simulink model "TPS_failure_system2020"  (R2020a)
settings: Solver=VariableStepAuto  StartTime=0.0  StopTime=10.0  RelTol=1e-3
undefined symbols (not defined in the file or in its folder): APP_modes
libraries: simulink x5
settings Model: Creator=Administrator  LastModifiedBy=Administrator

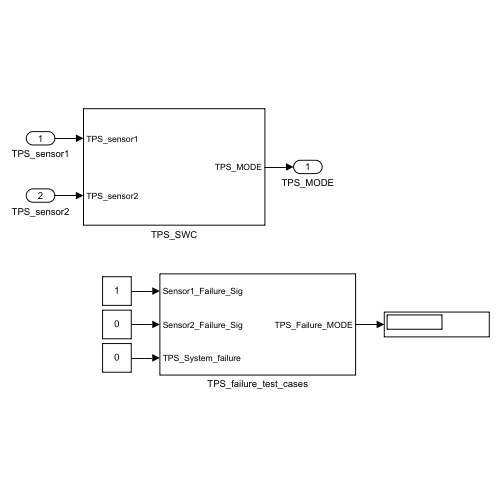
[thumbnail: Simulink's stored preview of the top-level diagram]
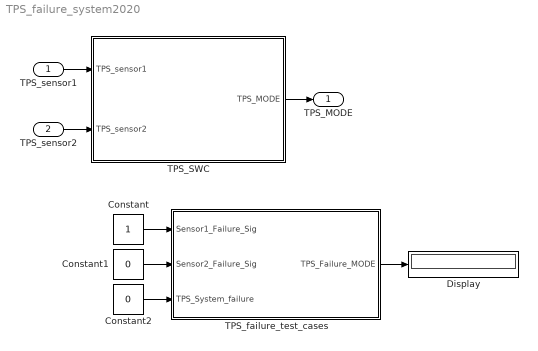
== system TPS_failure_system2020 ==
  TPS_sensor1 : Inport  OutDataTypeStr=single
  TPS_sensor2 : Inport  Port=2  OutDataTypeStr=single
  Constant : Constant  OutDataTypeStr=boolean
  Constant1 : Constant  Value=0  OutDataTypeStr=boolean
  Constant2 : Constant  Value=0  OutDataTypeStr=boolean
  Display : Display
  TPS_SWC : Subsystem
  TPS_failure_test_cases : Subsystem
  TPS_MODE : Outport
  wires:
  TPS_failure_test_cases/1(TPS_Failure_MODE) -> Display/1
  Constant/1 -> TPS_failure_test_cases/1(Sensor1_Failure_Sig)
  Constant1/1 -> TPS_failure_test_cases/2(Sensor2_Failure_Sig)
  Constant2/1 -> TPS_failure_test_cases/3(TPS_System_failure)
  TPS_SWC/1(TPS_MODE) -> TPS_MODE/1
  TPS_sensor1/1 -> TPS_SWC/1(TPS_sensor1)
  TPS_sensor2/1 -> TPS_SWC/2(TPS_sensor2)

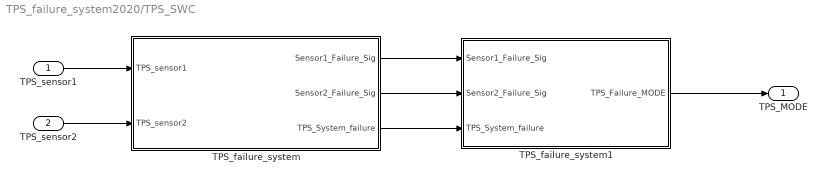
== system TPS_failure_system2020/TPS_SWC ==
  TPS_sensor1 : Inport  OutDataTypeStr=single
  TPS_sensor2 : Inport  Port=2  OutDataTypeStr=single
  TPS_failure_system : Subsystem
  TPS_failure_system1 : Subsystem
  TPS_MODE : Outport
  wires:
  TPS_failure_system/1(Sensor1_Failure_Sig) -> TPS_failure_system1/1(Sensor1_Failure_Sig)
  TPS_failure_system1/1(TPS_Failure_MODE) -> TPS_MODE/1
  TPS_sensor1/1 -> TPS_failure_system/1(TPS_sensor1)
  TPS_sensor2/1 -> TPS_failure_system/2(TPS_sensor2)
  TPS_failure_system/2(Sensor2_Failure_Sig) -> TPS_failure_system1/2(Sensor2_Failure_Sig)
  TPS_failure_system/3(TPS_System_failure) -> TPS_failure_system1/3(TPS_System_failure)

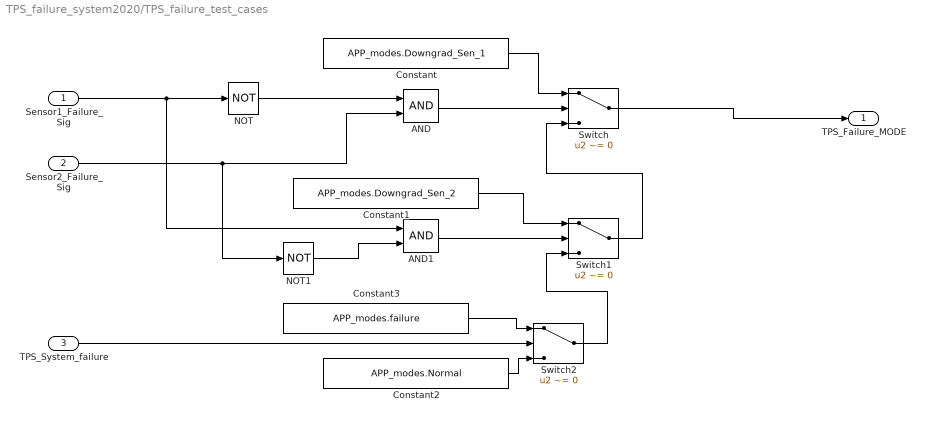
== system TPS_failure_system2020/TPS_failure_test_cases ==
  Sensor1_Failure_Sig : Inport  OutDataTypeStr=boolean
  Sensor2_Failure_Sig : Inport  Port=2  OutDataTypeStr=boolean
  TPS_System_failure : Inport  Port=3  OutDataTypeStr=boolean
  AND : Logic  AllPortsSameDT=off  OutDataTypeStr=boolean
  AND1 : Logic  AllPortsSameDT=off  OutDataTypeStr=boolean
  Constant : Constant  Value=APP_modes.Downgrad_Sen_1
  Constant1 : Constant  Value=APP_modes.Downgrad_Sen_2
  Constant2 : Constant  Value=APP_modes.Normal
  Constant3 : Constant  Value=APP_modes.failure
  NOT : Logic  Operator=NOT  IconShape=distinctive  AllPortsSameDT=off  OutDataTypeStr=boolean
  NOT1 : Logic  Operator=NOT  IconShape=distinctive  AllPortsSameDT=off  OutDataTypeStr=boolean
  Switch : Switch  Criteria=u2 ~= 0
  Switch1 : Switch  Criteria=u2 ~= 0
  Switch2 : Switch  Criteria=u2 ~= 0
  TPS_Failure_MODE : Outport
  wires:
  Switch/1 -> TPS_Failure_MODE/1
  Constant3/1 -> Switch2/1
  Switch2/1 -> Switch1/3
  Switch1/1 -> Switch/3
  Constant2/1 -> Switch2/3
  Constant1/1 -> Switch1/1
  Constant/1 -> Switch/1
  TPS_System_failure/1 -> Switch2/2
  AND1/1 -> Switch1/2
  AND/1 -> Switch/2
  NOT1/1 -> AND1/2
  Sensor1_Failure_Sig/1 -> NOT/1, AND1/1
  NOT/1 -> AND/1
  Sensor2_Failure_Sig/1 -> AND/2, NOT1/1

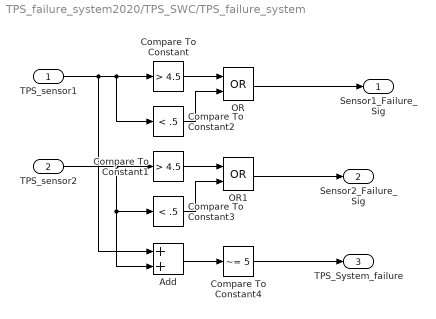
== system TPS_failure_system2020/TPS_SWC/TPS_failure_system ==
  TPS_sensor1 : Inport  OutDataTypeStr=single
  TPS_sensor2 : Inport  Port=2  OutDataTypeStr=single
  Add : Sum
  Compare To Constant : simulink/Logic and Bit Operations/Compare To Constant  relop=>  const=4.5  OutDataTypeStr=boolean
  Compare To Constant1 : simulink/Logic and Bit Operations/Compare To Constant  relop=>  const=4.5  OutDataTypeStr=boolean
  Compare To Constant2 : simulink/Logic and Bit Operations/Compare To Constant  relop=<  const=.5  OutDataTypeStr=boolean
  Compare To Constant3 : simulink/Logic and Bit Operations/Compare To Constant  relop=<  const=.5  OutDataTypeStr=boolean
  Compare To Constant4 : simulink/Logic and Bit Operations/Compare To Constant  relop=~=  const=5  OutDataTypeStr=boolean
  OR : Logic  Operator=OR  AllPortsSameDT=off  OutDataTypeStr=boolean
  OR1 : Logic  Operator=OR  AllPortsSameDT=off  OutDataTypeStr=boolean
  Sensor1_Failure_Sig : Outport  OutDataTypeStr=boolean
  Sensor2_Failure_Sig : Outport  Port=2  OutDataTypeStr=boolean
  TPS_System_failure : Outport  Port=3  OutDataTypeStr=boolean
  wires:
  Compare To Constant3/1 -> OR1/2
  Compare To Constant1/1 -> OR1/1
  OR1/1 -> Sensor2_Failure_Sig/1
  Compare To Constant/1 -> OR/1
  OR/1 -> Sensor1_Failure_Sig/1
  Add/1 -> Compare To Constant4/1
  TPS_sensor2/1 -> Compare To Constant3/1, Add/2, Compare To Constant1/1
  TPS_sensor1/1 -> Compare To Constant/1, Compare To Constant2/1, Add/1
  Compare To Constant4/1 -> TPS_System_failure/1
  Compare To Constant2/1 -> OR/2

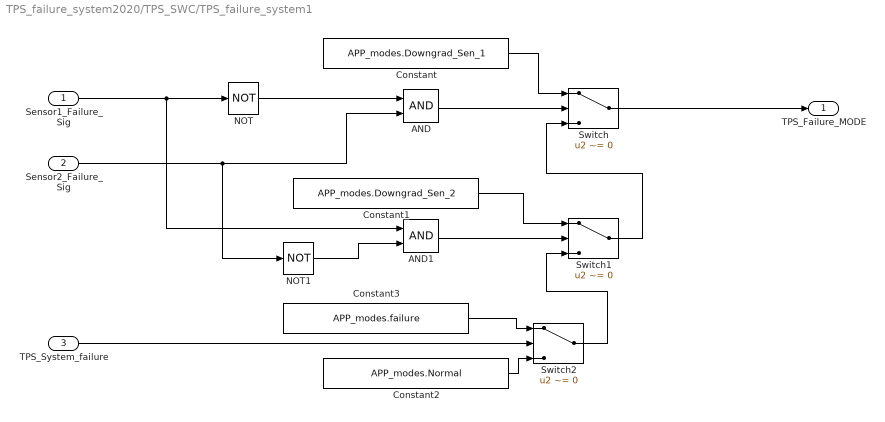
== system TPS_failure_system2020/TPS_SWC/TPS_failure_system1 ==
  Sensor1_Failure_Sig : Inport
  Sensor2_Failure_Sig : Inport  Port=2
  TPS_System_failure : Inport  Port=3
  AND : Logic  AllPortsSameDT=off  OutDataTypeStr=boolean
  AND1 : Logic  AllPortsSameDT=off  OutDataTypeStr=boolean
  Constant : Constant  Value=APP_modes.Downgrad_Sen_1
  Constant1 : Constant  Value=APP_modes.Downgrad_Sen_2
  Constant2 : Constant  Value=APP_modes.Normal
  Constant3 : Constant  Value=APP_modes.failure
  NOT : Logic  Operator=NOT  IconShape=distinctive  AllPortsSameDT=off  OutDataTypeStr=boolean
  NOT1 : Logic  Operator=NOT  IconShape=distinctive  AllPortsSameDT=off  OutDataTypeStr=boolean
  Switch : Switch  Criteria=u2 ~= 0
  Switch1 : Switch  Criteria=u2 ~= 0
  Switch2 : Switch  Criteria=u2 ~= 0
  TPS_Failure_MODE : Outport
  wires:
  Sensor2_Failure_Sig/1 -> NOT1/1, AND/2
  NOT/1 -> AND/1
  Sensor1_Failure_Sig/1 -> AND1/1, NOT/1
  NOT1/1 -> AND1/2
  AND/1 -> Switch/2
  AND1/1 -> Switch1/2
  TPS_System_failure/1 -> Switch2/2
  Constant/1 -> Switch/1
  Constant1/1 -> Switch1/1
  Constant2/1 -> Switch2/3
  Switch1/1 -> Switch/3
  Switch2/1 -> Switch1/3
  Constant3/1 -> Switch2/1
  Switch/1 -> TPS_Failure_MODE/1
